simulink subsystem "ContorlSeguidorDeLinea"  (R2023b)
settings: Solver=VariableStepAuto  StartTime=0.0  StopTime=10.0  RelTol=1e-3
libraries: arduinolib x2
settings Model: Creator=pablo  LastModifiedBy=pablo

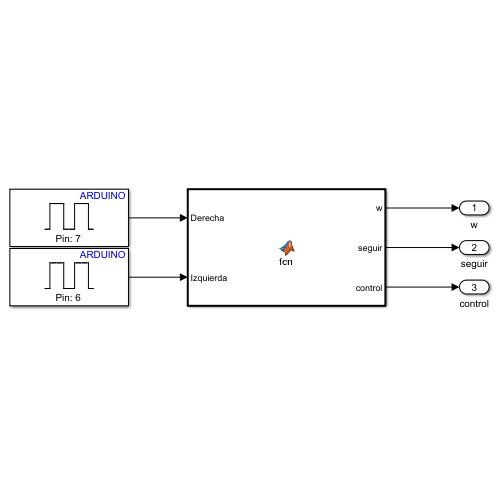
[thumbnail: Simulink's stored preview of the top-level diagram]
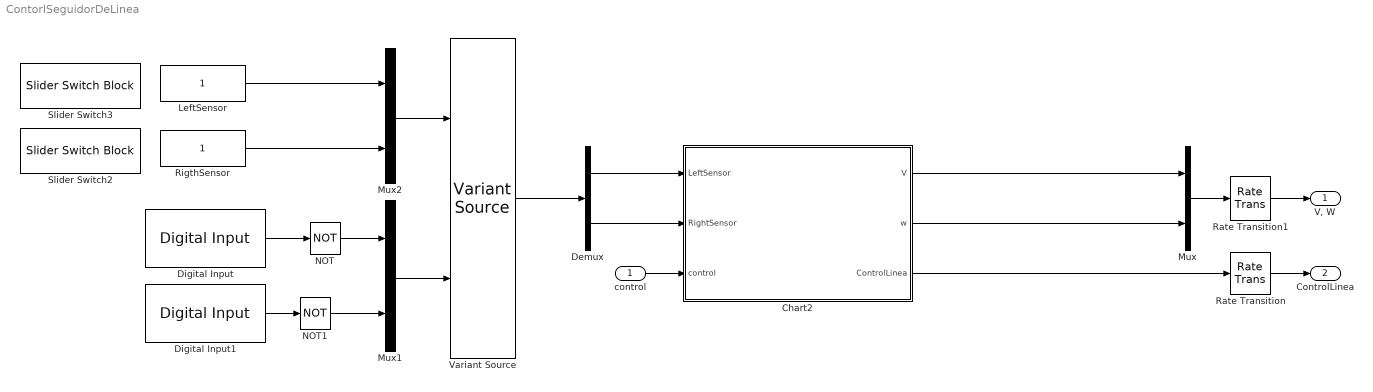
== system ContorlSeguidorDeLinea ==
  control : Inport
  Chart2 : Stateflow chart  TreatAsAtomicUnit=on
  Demux : Demux  Outputs=2
  Digital Input : arduinolib/Digital Input  pinNumber=6  mode=Default  Direction=input  SampleTime=0.01  blockPlatform=arduino
  Digital Input1 : arduinolib/Digital Input  pinNumber=7  mode=Default  Direction=input  SampleTime=0.01  blockPlatform=arduino
  LeftSensor : Constant
  Mux : Mux  Inputs=2
  Mux1 : Mux  Inputs=2
  Mux2 : Mux  Inputs=2
  NOT : Logic  Operator=NOT  IconShape=distinctive  AllPortsSameDT=off  OutDataTypeStr=boolean
  NOT1 : Logic  Operator=NOT  IconShape=distinctive  AllPortsSameDT=off  OutDataTypeStr=boolean
  Rate Transition : RateTransition
  Rate Transition1 : RateTransition
  RigthSensor : Constant
  Slider Switch2 : SliderSwitchBlock
      settings: Values={{'Linea', 'NoLinea'}, [1 0]}
  Slider Switch3 : SliderSwitchBlock
      settings: Values={{'Linea', 'NoLinea'}, [1 0]}
  Variant Source : VariantSource  VariantControlMode=sim codegen switching
  "V, W" : Outport
  ControlLinea : Outport  Port=2  OutDataTypeStr=double
  wires:
  Chart2/3(ControlLinea) -> Rate Transition/1
  Demux/1 -> Chart2/1(LeftSensor)
  Demux/2 -> Chart2/2(RightSensor)
  Chart2/1(V) -> Mux/1
  Mux/1 -> Rate Transition1/1
  Rate Transition1/1 -> "V, W"/1
  Rate Transition/1 -> ControlLinea/1
  control/1 -> Chart2/3(control)
  RigthSensor/1 -> Mux2/2
  LeftSensor/1 -> Mux2/1
  Mux2/1 -> Variant Source/1
  Digital Input1/1 -> NOT1/1
  Digital Input/1 -> NOT/1
  NOT/1 -> Mux1/1
  NOT1/1 -> Mux1/2
  Mux1/1 -> Variant Source/2
  Variant Source/1 -> Demux/1
  Chart2/2(w) -> Mux/2

== stateflow chart ContorlSeguidorDeLinea/Chart2 ==
  state Transicion_Parar
  state ObstaculoIzq
    en:
    ControlLinea = 1;
    V = 0.150;
    w = -1.5;
  state ObstaculoDcha
    en:
    ControlLinea = 1;
    V = 0.150;
    w = 1.5;
  state Seguir
    en:
    ControlLinea = 1;
    V = 0.150;
    w = 0;
  state PreparadoParabuscarLinea
  state NoSeguir
    en:
    after(2,sec)
    ControlLinea = 0;
    V = 0.150;
    w = 0;
  state BuscarLinea
    en:
    ControlLinea = 1;
    V = 0.150;
    w = 0;
  state Transicion_Empezar
  Transicion_Parar -> NoSeguir : after(0.75,sec)
  ObstaculoDcha -> Transicion_Parar [order 2] : [RightSensor==0 & LeftSensor==0 & ControlLinea == 1]
  ObstaculoIzq -> Transicion_Parar [order 2] : [RightSensor==0 & LeftSensor==0 & ControlLinea == 1]
  Seguir -> Transicion_Parar [order 1] : [RightSensor==0 & LeftSensor==0 & ControlLinea == 1]
  Seguir -> ObstaculoIzq [order 3] : [LeftSensor==0]
  Seguir -> ObstaculoDcha [order 2] : [RightSensor==0]
  ObstaculoIzq -> PreparadoParabuscarLinea [order 3] : [control == 1]
  PreparadoParabuscarLinea -> BuscarLinea : [control == 0]
  BuscarLinea -> PreparadoParabuscarLinea [order 3] : [control == 1]
  ObstaculoDcha -> PreparadoParabuscarLinea [order 3] : [control == 1]
  Seguir -> PreparadoParabuscarLinea [order 4] : [control == 1]
  (default) -> NoSeguir
  ObstaculoIzq -> Seguir [order 1] : [LeftSensor==1]
  ObstaculoDcha -> Seguir [order 1] : [RightSensor==1]
  Transicion_Empezar -> Seguir : after(0.75,sec)
  BuscarLinea -> NoSeguir [order 2] : after(5,sec)
  NoSeguir -> Transicion_Empezar : [RightSensor==0 & LeftSensor==0 & ControlLinea == 0]
  BuscarLinea -> Transicion_Empezar [order 1] : [RightSensor==0 || LeftSensor==0]
  data: V output double size=1; w output double size=1; LeftSensor input size=1; RightSensor input size=1; ControlLinea output double size=1; control input
  data V settings: description=Velocidad lineal del vehiculo
